simulink library "NHR9400"  (R2020b)
settings: Solver=VariableStepAuto  StartTime=0.0  StopTime=10.0  RelTol=1e-3
undefined symbols (not defined in the file or in its folder): Ts
libraries: simulink x31, fl_lib x19, nesl_utility x12, powerlib_meascontrol x9
settings Model: Creator=argol  LastModifiedBy=argol

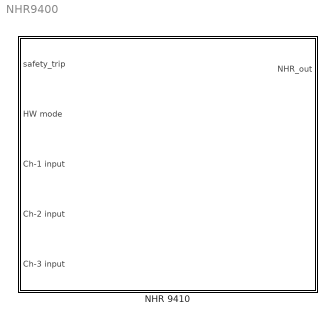
== system NHR9400 ==
  NHR 9410 : Subsystem  mask{p_switch=1, VslewAC=0.0, FslewAC=500.0, VslewDC=0.0, IslewDC=0.0, PslewDC=0.0}
      mask prompts: p_switch "Enter 1 to turn ON, 0 to turn OFF NHR 9410"
      mask DialogControl DescTextVar Prompt: NHR 9410
      mask DialogControl Container3 Prompt: Slew Rates
      mask DialogControl Control2 Prompt: AC Voltage slew rate [0-500000V/s]:
      mask DialogControl f Prompt: Frequency slew rate [0-500 /s]
      mask DialogControl Control3 Prompt: DC Voltage slew rate [0-20000V/s]:
      mask DialogControl Control4 Prompt: DC current slew rate [0-100000A/s]:
      mask DialogControl Control5 Prompt: DC power slew rate [0-1000000W/s]:
      mask Display: image('NHR9410.png');

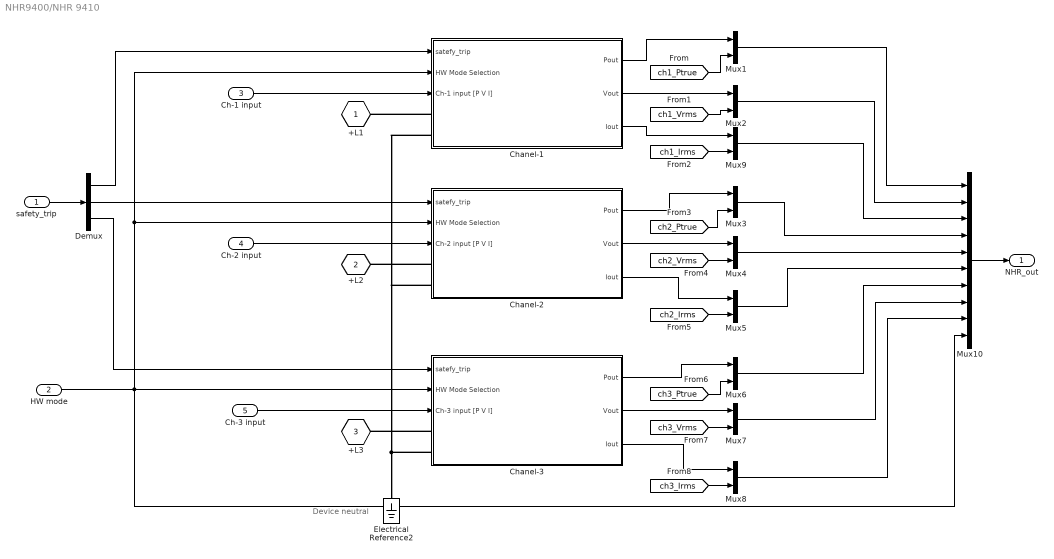
== system NHR9400/NHR 9410 ==
  note: Device neutral
  safety_trip : Inport
  HW mode : Inport  Port=2
  Ch-1 input : Inport  Port=3
  Ch-2 input : Inport  Port=4
  Ch-3 input : Inport  Port=5
  Chanel-1 : Subsystem
  Chanel-2 : Subsystem
  Chanel-3 : Subsystem
  Demux : Demux  Outputs=3
  Electrical Reference2 : fl_lib/Electrical/Electrical Elements/Electrical Reference
  Mux{1..9} (9 alike) : Mux  Inputs=2
  Mux10 : Mux  Inputs=10
  +L1 : PMIOPort  Side=Right
  +L2 : PMIOPort  Port=2  Side=Right
  +L3 : PMIOPort  Port=3  Side=Right
  NHR_out : Outport  VectorParamsAs1DForOutWhenUnconnected=off
  wires:
  Ch-3 input/1 -> Chanel-3/3(Ch-3 input [P V I])
  Ch-1 input/1 -> Chanel-1/3(Ch-1 input [P V I])
  Ch-2 input/1 -> Chanel-2/3(Ch-2 input [P V I])
  Chanel-2/1(Pout) -> Mux3/1
  Chanel-2/2(Vout) -> Mux4/1
  Chanel-2/3(Iout) -> Mux5/1
  Chanel-3/1(Pout) -> Mux6/1
  Chanel-3/2(Vout) -> Mux7/1
  Chanel-3/3(Iout) -> Mux8/1
  [ch2_Ptrue] -> Mux3/2
  [ch2_Vrms] -> Mux4/2
  [ch2_Irms] -> Mux5/2
  [ch3_Ptrue] -> Mux6/2
  [ch3_Vrms] -> Mux7/2
  [ch3_Irms] -> Mux8/2
  Mux1/1 -> Mux10/1
  Mux2/1 -> Mux10/2
  Mux9/1 -> Mux10/3
  Mux3/1 -> Mux10/4
  Mux4/1 -> Mux10/5
  Mux6/1 -> Mux10/7
  Mux7/1 -> Mux10/8
  Mux8/1 -> Mux10/9
  Demux/2 -> Chanel-2/1(satefy_trip)
  Demux/1 -> Chanel-1/1(satefy_trip)
  safety_trip/1 -> Demux/1
  Demux/3 -> Chanel-3/1(satefy_trip)
  Mux5/1 -> Mux10/6
  HW mode/1 -> Chanel-2/2(HW Mode Selection), Chanel-1/2(HW Mode Selection), Mux10/10, Chanel-3/2(HW Mode Selection)
  Mux10/1 -> NHR_out/1
  Chanel-1/2(Vout) -> Mux2/1
  Chanel-1/1(Pout) -> Mux1/1
  Chanel-1/3(Iout) -> Mux9/1
  [ch1_Ptrue] -> Mux1/2
  [ch1_Vrms] -> Mux2/2
  [ch1_Irms] -> Mux9/2
  connections:
  Chanel-1/LConn1 -- +L1/RConn1
  Chanel-2/LConn1 -- +L2/RConn1
  Chanel-3/LConn1 -- +L3/RConn1
  Chanel-3/LConn2 -- Chanel-1/LConn2 -- Chanel-2/LConn2 -- Electrical Reference2/LConn1

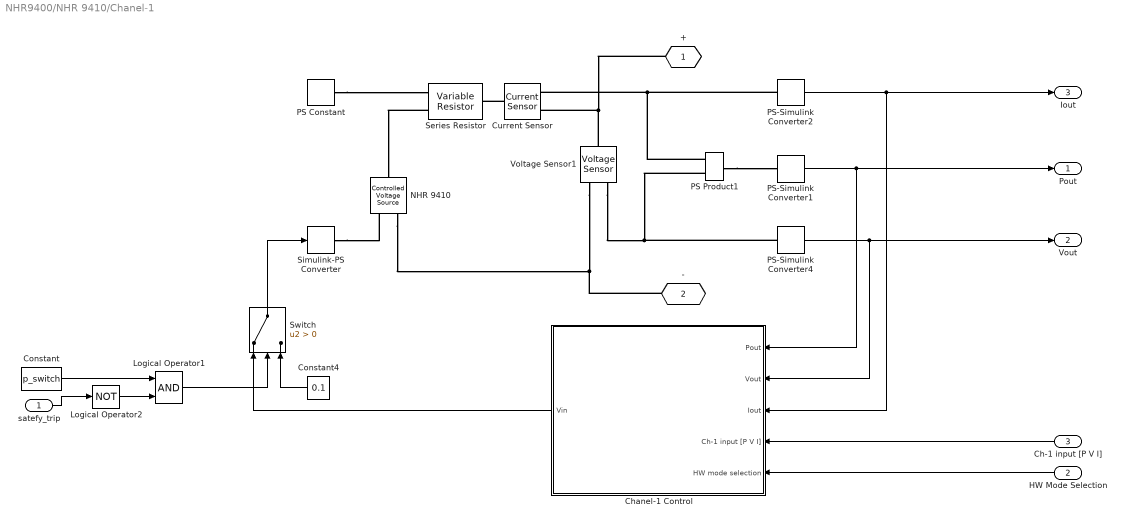
== system NHR9400/NHR 9410/Chanel-1 ==
  satefy_trip : Inport
  HW Mode Selection : Inport  Port=2
  Ch-1 input [P V I] : Inport  Port=3
  Chanel-1 Control : Subsystem
  Constant : Constant  Value=p_switch
  Constant4 : Constant  Value=0.1
  Current Sensor : fl_lib/Electrical/Electrical Sensors/Current Sensor
  Logical Operator1 : Logic  AllPortsSameDT=off  OutDataTypeStr=boolean
  Logical Operator2 : Logic  Operator=NOT  AllPortsSameDT=off  OutDataTypeStr=boolean
  NHR 9410 : fl_lib/Electrical/Electrical Sources/Controlled Voltage Source
  PS Constant : fl_lib/Physical Signals/Sources/PS Constant  constant=0
  PS Product1 : fl_lib/Physical Signals/Functions/PS Product
  PS-Simulink Converter1 : nesl_utility/PS-Simulink Converter  PhysicalDomain=network_engine_domain  SubClassName=ps_output  LeftPortType=input  RightPortType=output  PseudoPeriodic=off  Frequencies=[]  Unit=inherit  AffineConversion=off
  PS-Simulink Converter2 : nesl_utility/PS-Simulink Converter  PhysicalDomain=network_engine_domain  SubClassName=ps_output  LeftPortType=input  RightPortType=output  PseudoPeriodic=off  Frequencies=[]  Unit=1  AffineConversion=off
  PS-Simulink Converter4 : nesl_utility/PS-Simulink Converter  PhysicalDomain=network_engine_domain  SubClassName=ps_output  LeftPortType=input  RightPortType=output  PseudoPeriodic=off  Frequencies=[]  Unit=1  AffineConversion=off
  Series Resistor : fl_lib/Electrical/Electrical Elements/Variable Resistor  Rmin=0.0001 Ohm  i_specify=off  i_priority=None  i=0 A  i_nominal_specify=off  i_nominal_unit=A  i_nominal_value=1  v_specify=off  v_priority=None  v=0 V  v_nominal_specify=off  v_nominal_unit=V  v_nominal_value=1
  Simulink-PS Converter : nesl_utility/Simulink-PS Converter  PhysicalDomain=network_engine_domain  SubClassName=ps_input  LeftPortType=input  RightPortType=output  PseudoPeriodic=off  Frequencies=[]  NoiseDistribution=none  NoiseParameters=[]  Unit=1  AffineConversion=off  FilteringAndDerivatives=filter  SimscapeFilterOrder=1  InputFilterTimeConstant=0.001  UdotUserProvided=0
  Switch : Switch  Criteria=u2 > Threshold  ZeroCross=off
  Voltage Sensor1 : fl_lib/Electrical/Electrical Sensors/Voltage Sensor
  + : PMIOPort  Tag=PMCPort  Side=Left
  - : PMIOPort  Tag=PMCPort  Port=2  Side=Left
  Pout : Outport  VectorParamsAs1DForOutWhenUnconnected=off
  Vout : Outport  Port=2  VectorParamsAs1DForOutWhenUnconnected=off
  Iout : Outport  Port=3  VectorParamsAs1DForOutWhenUnconnected=off
  wires:
  Constant/1 -> Logical Operator1/1
  satefy_trip/1 -> Logical Operator2/1
  Logical Operator2/1 -> Logical Operator1/2
  Switch/1 -> Simulink-PS Converter/1
  Chanel-1 Control/1(Vin) -> Switch/1
  Constant4/1 -> Switch/3
  Logical Operator1/1 -> Switch/2
  PS-Simulink Converter2/1 -> Iout/1, Chanel-1 Control/3(Iout)
  PS-Simulink Converter4/1 -> Vout/1, Chanel-1 Control/2(Vout)
  PS-Simulink Converter1/1 -> Pout/1, Chanel-1 Control/1(Pout)
  HW Mode Selection/1 -> Chanel-1 Control/5(HW mode selection)
  Ch-1 input [P V I]/1 -> Chanel-1 Control/4(Ch-1 input [P V I])
  connections:
  Current Sensor/LConn1 -- Series Resistor/RConn1
  PS Constant/RConn1 -- Series Resistor/LConn1
  PS Product1/RConn1 -- PS-Simulink Converter1/LConn1
  Series Resistor/LConn2 -- NHR 9410/LConn1
  Simulink-PS Converter/RConn1 -- NHR 9410/RConn1
  Voltage Sensor1/LConn1 -- +/RConn1 -- Current Sensor/RConn2
  PS-Simulink Converter2/LConn1 -- PS Product1/LConn1 -- Current Sensor/RConn1
  NHR 9410/RConn2 -- -/RConn1 -- Voltage Sensor1/RConn2
  Voltage Sensor1/RConn1 -- PS Product1/LConn2 -- PS-Simulink Converter4/LConn1

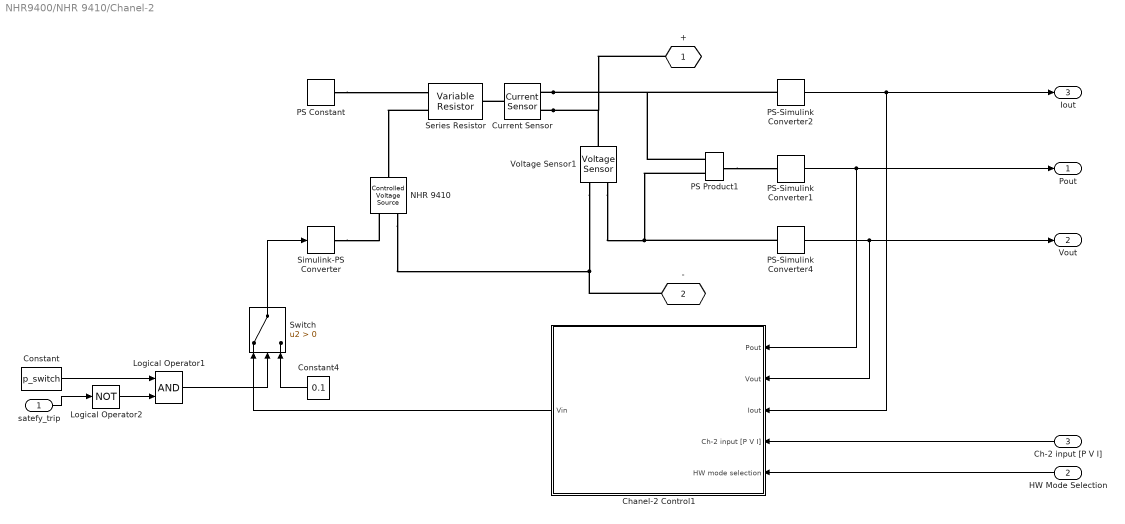
== system NHR9400/NHR 9410/Chanel-2 ==
  satefy_trip : Inport
  HW Mode Selection : Inport  Port=2
  Ch-2 input [P V I] : Inport  Port=3
  Chanel-2 Control1 : Subsystem
  Constant : Constant  Value=p_switch
  Constant4 : Constant  Value=0.1
  Current Sensor : fl_lib/Electrical/Electrical Sensors/Current Sensor
  Logical Operator1 : Logic  AllPortsSameDT=off  OutDataTypeStr=boolean
  Logical Operator2 : Logic  Operator=NOT  AllPortsSameDT=off  OutDataTypeStr=boolean
  NHR 9410 : fl_lib/Electrical/Electrical Sources/Controlled Voltage Source
  PS Constant : fl_lib/Physical Signals/Sources/PS Constant  constant=0
  PS Product1 : fl_lib/Physical Signals/Functions/PS Product
  PS-Simulink Converter1 : nesl_utility/PS-Simulink Converter  PhysicalDomain=network_engine_domain  SubClassName=ps_output  LeftPortType=input  RightPortType=output  PseudoPeriodic=off  Frequencies=[]  Unit=inherit  AffineConversion=off
  PS-Simulink Converter2 : nesl_utility/PS-Simulink Converter  PhysicalDomain=network_engine_domain  SubClassName=ps_output  LeftPortType=input  RightPortType=output  PseudoPeriodic=off  Frequencies=[]  Unit=1  AffineConversion=off
  PS-Simulink Converter4 : nesl_utility/PS-Simulink Converter  PhysicalDomain=network_engine_domain  SubClassName=ps_output  LeftPortType=input  RightPortType=output  PseudoPeriodic=off  Frequencies=[]  Unit=1  AffineConversion=off
  Series Resistor : fl_lib/Electrical/Electrical Elements/Variable Resistor  Rmin=0.0001 Ohm  i_specify=off  i_priority=None  i=0 A  i_nominal_specify=off  i_nominal_unit=A  i_nominal_value=1  v_specify=off  v_priority=None  v=0 V  v_nominal_specify=off  v_nominal_unit=V  v_nominal_value=1
  Simulink-PS Converter : nesl_utility/Simulink-PS Converter  PhysicalDomain=network_engine_domain  SubClassName=ps_input  LeftPortType=input  RightPortType=output  PseudoPeriodic=off  Frequencies=[]  NoiseDistribution=none  NoiseParameters=[]  Unit=1  AffineConversion=off  FilteringAndDerivatives=filter  SimscapeFilterOrder=1  InputFilterTimeConstant=0.001  UdotUserProvided=0
  Switch : Switch  Criteria=u2 > Threshold  ZeroCross=off
  Voltage Sensor1 : fl_lib/Electrical/Electrical Sensors/Voltage Sensor
  + : PMIOPort  Tag=PMCPort  Side=Left
  - : PMIOPort  Tag=PMCPort  Port=2  Side=Left
  Pout : Outport  VectorParamsAs1DForOutWhenUnconnected=off
  Vout : Outport  Port=2  VectorParamsAs1DForOutWhenUnconnected=off
  Iout : Outport  Port=3  VectorParamsAs1DForOutWhenUnconnected=off
  wires:
  Ch-2 input [P V I]/1 -> Chanel-2 Control1/4(Ch-2 input [P V I])
  HW Mode Selection/1 -> Chanel-2 Control1/5(HW mode selection)
  PS-Simulink Converter1/1 -> Chanel-2 Control1/1(Pout), Pout/1
  PS-Simulink Converter4/1 -> Chanel-2 Control1/2(Vout), Vout/1
  PS-Simulink Converter2/1 -> Chanel-2 Control1/3(Iout), Iout/1
  Logical Operator1/1 -> Switch/2
  Constant4/1 -> Switch/3
  Chanel-2 Control1/1(Vin) -> Switch/1
  Switch/1 -> Simulink-PS Converter/1
  Logical Operator2/1 -> Logical Operator1/2
  satefy_trip/1 -> Logical Operator2/1
  Constant/1 -> Logical Operator1/1
  connections:
  PS-Simulink Converter4/LConn1 -- PS Product1/LConn2 -- Voltage Sensor1/RConn1
  Voltage Sensor1/RConn2 -- -/RConn1 -- NHR 9410/RConn2
  Current Sensor/RConn1 -- PS Product1/LConn1 -- PS-Simulink Converter2/LConn1
  Current Sensor/RConn2 -- +/RConn1 -- Voltage Sensor1/LConn1
  Simulink-PS Converter/RConn1 -- NHR 9410/RConn1
  Series Resistor/LConn2 -- NHR 9410/LConn1
  PS Product1/RConn1 -- PS-Simulink Converter1/LConn1
  PS Constant/RConn1 -- Series Resistor/LConn1
  Current Sensor/LConn1 -- Series Resistor/RConn1

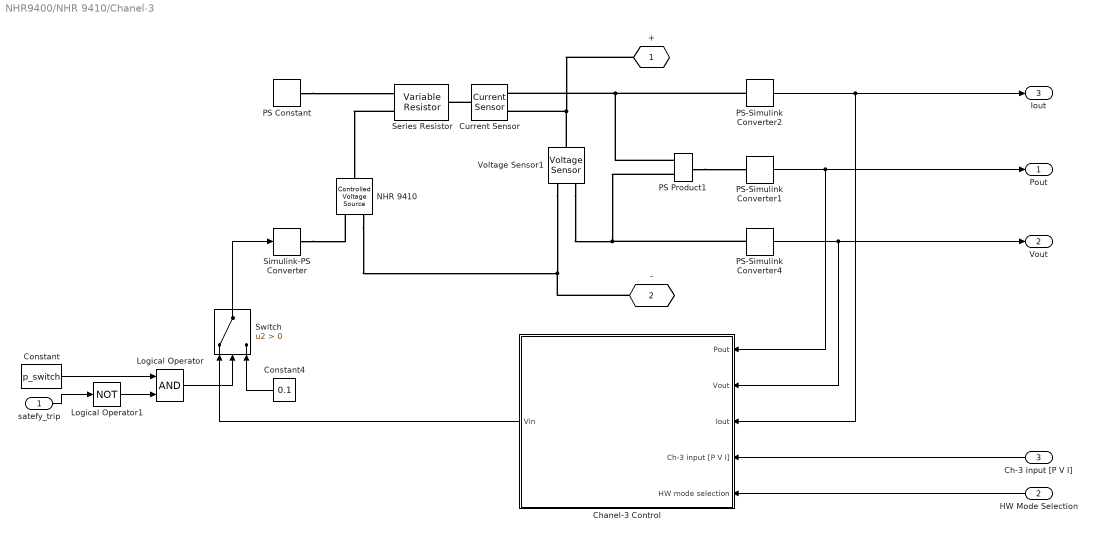
== system NHR9400/NHR 9410/Chanel-3 ==
  satefy_trip : Inport
  HW Mode Selection : Inport  Port=2
  Ch-3 input [P V I] : Inport  Port=3
  Chanel-3 Control : Subsystem
  Constant : Constant  Value=p_switch
  Constant4 : Constant  Value=0.1
  Current Sensor : fl_lib/Electrical/Electrical Sensors/Current Sensor
  Logical Operator : Logic  AllPortsSameDT=off  OutDataTypeStr=boolean
  Logical Operator1 : Logic  Operator=NOT  AllPortsSameDT=off  OutDataTypeStr=boolean
  NHR 9410 : fl_lib/Electrical/Electrical Sources/Controlled Voltage Source
  PS Constant : fl_lib/Physical Signals/Sources/PS Constant  constant=0
  PS Product1 : fl_lib/Physical Signals/Functions/PS Product
  PS-Simulink Converter1 : nesl_utility/PS-Simulink Converter  PhysicalDomain=network_engine_domain  SubClassName=ps_output  LeftPortType=input  RightPortType=output  PseudoPeriodic=off  Frequencies=[]  Unit=inherit  AffineConversion=off
  PS-Simulink Converter2 : nesl_utility/PS-Simulink Converter  PhysicalDomain=network_engine_domain  SubClassName=ps_output  LeftPortType=input  RightPortType=output  PseudoPeriodic=off  Frequencies=[]  Unit=1  AffineConversion=off
  PS-Simulink Converter4 : nesl_utility/PS-Simulink Converter  PhysicalDomain=network_engine_domain  SubClassName=ps_output  LeftPortType=input  RightPortType=output  PseudoPeriodic=off  Frequencies=[]  Unit=1  AffineConversion=off
  Series Resistor : fl_lib/Electrical/Electrical Elements/Variable Resistor  Rmin=0.0001 Ohm  i_specify=off  i_priority=None  i=0 A  i_nominal_specify=off  i_nominal_unit=A  i_nominal_value=1  v_specify=off  v_priority=None  v=0 V  v_nominal_specify=off  v_nominal_unit=V  v_nominal_value=1
  Simulink-PS Converter : nesl_utility/Simulink-PS Converter  PhysicalDomain=network_engine_domain  SubClassName=ps_input  LeftPortType=input  RightPortType=output  PseudoPeriodic=off  Frequencies=[]  NoiseDistribution=none  NoiseParameters=[]  Unit=1  AffineConversion=off  FilteringAndDerivatives=filter  SimscapeFilterOrder=1  InputFilterTimeConstant=0.001  UdotUserProvided=0
  Switch : Switch  Criteria=u2 > Threshold  ZeroCross=off
  Voltage Sensor1 : fl_lib/Electrical/Electrical Sensors/Voltage Sensor
  + : PMIOPort  Tag=PMCPort  Side=Left
  - : PMIOPort  Tag=PMCPort  Port=2  Side=Left
  Pout : Outport  VectorParamsAs1DForOutWhenUnconnected=off
  Vout : Outport  Port=2  VectorParamsAs1DForOutWhenUnconnected=off
  Iout : Outport  Port=3  VectorParamsAs1DForOutWhenUnconnected=off
  wires:
  PS-Simulink Converter2/1 -> Iout/1, Chanel-3 Control/3(Iout)
  PS-Simulink Converter4/1 -> Vout/1, Chanel-3 Control/2(Vout)
  PS-Simulink Converter1/1 -> Pout/1, Chanel-3 Control/1(Pout)
  HW Mode Selection/1 -> Chanel-3 Control/5(HW mode selection)
  Ch-3 input [P V I]/1 -> Chanel-3 Control/4(Ch-3 input [P V I])
  Constant4/1 -> Switch/3
  Chanel-3 Control/1(Vin) -> Switch/1
  Switch/1 -> Simulink-PS Converter/1
  Logical Operator1/1 -> Logical Operator/2
  satefy_trip/1 -> Logical Operator1/1
  Constant/1 -> Logical Operator/1
  Logical Operator/1 -> Switch/2
  connections:
  Current Sensor/LConn1 -- Series Resistor/RConn1
  PS Constant/RConn1 -- Series Resistor/LConn1
  PS Product1/RConn1 -- PS-Simulink Converter1/LConn1
  Series Resistor/LConn2 -- NHR 9410/LConn1
  Simulink-PS Converter/RConn1 -- NHR 9410/RConn1
  Voltage Sensor1/LConn1 -- +/RConn1 -- Current Sensor/RConn2
  PS-Simulink Converter2/LConn1 -- PS Product1/LConn1 -- Current Sensor/RConn1
  NHR 9410/RConn2 -- -/RConn1 -- Voltage Sensor1/RConn2
  Voltage Sensor1/RConn1 -- PS Product1/LConn2 -- PS-Simulink Converter4/LConn1

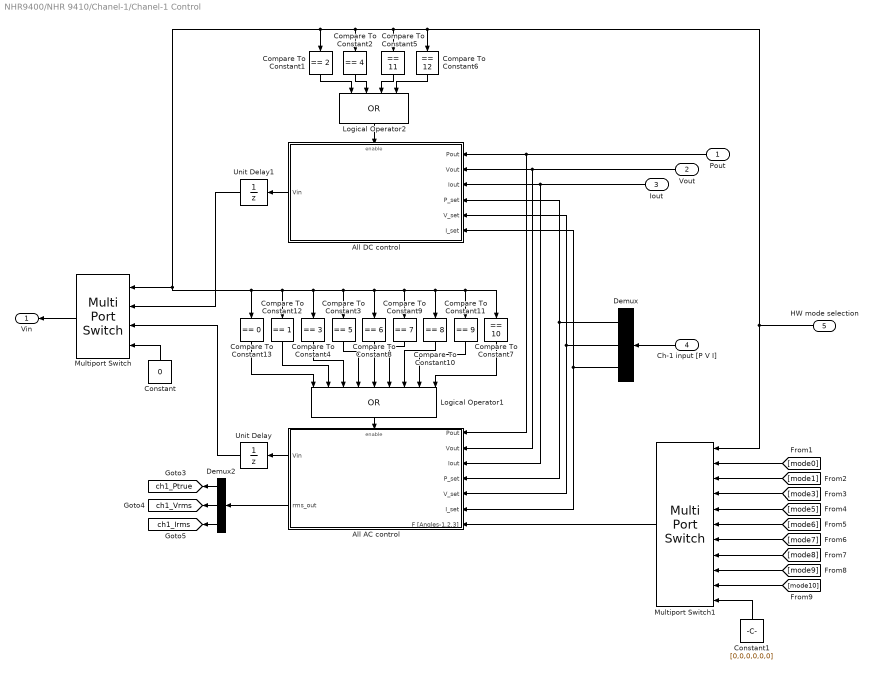
== system NHR9400/NHR 9410/Chanel-1/Chanel-1 Control ==
  Pout : Inport
  Vout : Inport  Port=2
  Iout : Inport  Port=3
  Ch-1 input [P V I] : Inport  Port=4
  HW mode selection : Inport  Port=5
  All AC control : Subsystem
      settings: MinAlgLoopOccurrences=on
  All DC control : Subsystem
      settings: MinAlgLoopOccurrences=on
  Compare To Constant1 : simulink/Logic and Bit Operations/Compare To Constant  relop===  const=2  OutDataTypeStr=boolean
  Compare To Constant10 : simulink/Logic and Bit Operations/Compare To Constant  relop===  const=8  OutDataTypeStr=boolean
  Compare To Constant11 : simulink/Logic and Bit Operations/Compare To Constant  relop===  const=9  OutDataTypeStr=boolean
  Compare To Constant12 : simulink/Logic and Bit Operations/Compare To Constant  relop===  const=1  OutDataTypeStr=boolean
  Compare To Constant13 : simulink/Logic and Bit Operations/Compare To Constant  relop===  const=0  OutDataTypeStr=boolean
  Compare To Constant2 : simulink/Logic and Bit Operations/Compare To Constant  relop===  const=4  OutDataTypeStr=boolean
  Compare To Constant3 : simulink/Logic and Bit Operations/Compare To Constant  relop===  const=5  OutDataTypeStr=boolean
  Compare To Constant4 : simulink/Logic and Bit Operations/Compare To Constant  relop===  const=3  OutDataTypeStr=boolean
  Compare To Constant5 : simulink/Logic and Bit Operations/Compare To Constant  relop===  const=11  OutDataTypeStr=boolean
  Compare To Constant6 : simulink/Logic and Bit Operations/Compare To Constant  relop===  const=12  OutDataTypeStr=boolean
  Compare To Constant7 : simulink/Logic and Bit Operations/Compare To Constant  relop===  const=10  OutDataTypeStr=boolean
  Compare To Constant8 : simulink/Logic and Bit Operations/Compare To Constant  relop===  const=6  OutDataTypeStr=boolean
  Compare To Constant9 : simulink/Logic and Bit Operations/Compare To Constant  relop===  const=7  OutDataTypeStr=boolean
  Constant : Constant  Value=0
  Constant1 : Constant  Value=[0,0,0,0,0,0]
  Demux : Demux  Outputs=3
  Demux2 : Demux  Outputs=3
  Logical Operator1 : Logic  Operator=OR  Inputs=9  AllPortsSameDT=off  OutDataTypeStr=boolean
  Logical Operator2 : Logic  Operator=OR  Inputs=4  AllPortsSameDT=off  OutDataTypeStr=boolean
  Multiport Switch : MultiPortSwitch  DataPortOrder=Specify indices  Inputs=13  DataPortIndices={[2,4,11,12],[0,1,3,5,6,7,8,9,10]}  DataPortForDefault=Additional data port  DiagnosticForDefault=None
  Multiport Switch1 : MultiPortSwitch  DataPortOrder=Specify indices  Inputs=13  DataPortIndices={0,1,3,5,6,7,8,9,10}  DataPortForDefault=Additional data port  DiagnosticForDefault=None
  Unit Delay : UnitDelay  SampleTime=-1  HasFrameUpgradeWarning=on
  Unit Delay1 : UnitDelay  SampleTime=-1  HasFrameUpgradeWarning=on
  Vin : Outport  VectorParamsAs1DForOutWhenUnconnected=off
  tag scope: ch1_Irms=global, ch1_Ptrue=global, ch1_Vrms=global
  wires:
  Compare To Constant2/1 -> Logical Operator2/2
  Compare To Constant1/1 -> Logical Operator2/1
  HW mode selection/1 -> Multiport Switch1/1, Compare To Constant6/1, Compare To Constant5/1, Compare To Constant2/1, Compare To Constant1/1, Multiport Switch/1, Compare To Constant13/1, Compare To Constant12/1, Compare To Constant3/1, Compare To Constant7/1, Compare To Constant11/1, Compare To Constant10/1, Compare To Constant9/1, Compare To Constant8/1, Compare To Constant4/1
  All AC control/1(Vin) -> Unit Delay/1
  All DC control/1(Vin) -> Unit Delay1/1
  All AC control/2(rms_out) -> Demux2/1
  Logical Operator1/1 -> All AC control/Enable
  Logical Operator2/1 -> All DC control/Enable
  Constant/1 -> Multiport Switch/4
  Multiport Switch/1 -> Vin/1
  Pout/1 -> All DC control/1(Pout), All AC control/1(Pout)
  Iout/1 -> All DC control/3(Iout), All AC control/3(Iout)
  Demux2/1 -> [ch1_Ptrue]
  Demux2/3 -> [ch1_Irms]
  Demux2/2 -> [ch1_Vrms]
  Vout/1 -> All DC control/2(Vout), All AC control/2(Vout)
  Ch-1 input [P V I]/1 -> Demux/1
  Demux/1 -> All AC control/4(P_set), All DC control/4(P_set)
  Demux/2 -> All AC control/5(V_set), All DC control/5(V_set)
  Demux/3 -> All AC control/6(I_set), All DC control/6(I_set)
  Compare To Constant5/1 -> Logical Operator2/3
  Compare To Constant6/1 -> Logical Operator2/4
  Compare To Constant8/1 -> Logical Operator1/5
  Compare To Constant9/1 -> Logical Operator1/6
  Compare To Constant10/1 -> Logical Operator1/7
  Compare To Constant11/1 -> Logical Operator1/8
  Compare To Constant7/1 -> Logical Operator1/9
  Compare To Constant13/1 -> Logical Operator1/1
  Compare To Constant12/1 -> Logical Operator1/2
  Compare To Constant4/1 -> Logical Operator1/3
  Compare To Constant3/1 -> Logical Operator1/4
  [mode0] -> Multiport Switch1/2
  [mode1] -> Multiport Switch1/3
  [mode3] -> Multiport Switch1/4
  [mode5] -> Multiport Switch1/5
  [mode6] -> Multiport Switch1/6
  [mode7] -> Multiport Switch1/7
  [mode8] -> Multiport Switch1/8
  [mode9] -> Multiport Switch1/9
  [mode10] -> Multiport Switch1/10
  Constant1/1 -> Multiport Switch1/11
  Multiport Switch1/1 -> All AC control/7(F [Angles-1,2,3])
  Unit Delay/1 -> Multiport Switch/3
  Unit Delay1/1 -> Multiport Switch/2

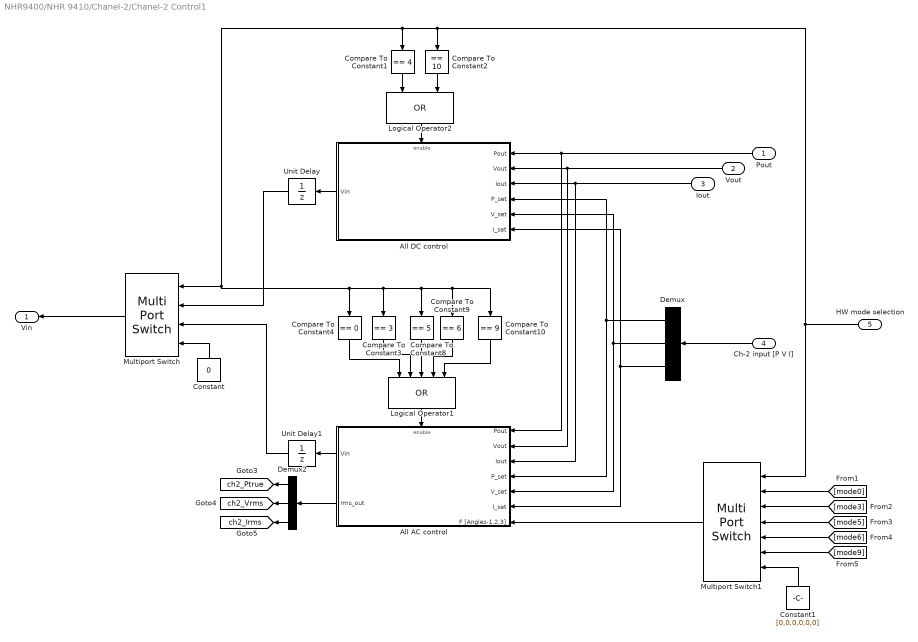
== system NHR9400/NHR 9410/Chanel-2/Chanel-2 Control1 ==
  Pout : Inport
  Vout : Inport  Port=2
  Iout : Inport  Port=3
  Ch-2 input [P V I] : Inport  Port=4
  HW mode selection : Inport  Port=5
  All AC control : Subsystem
      settings: MinAlgLoopOccurrences=on
  All DC control : Subsystem
      settings: MinAlgLoopOccurrences=on
  Compare To Constant1 : simulink/Logic and Bit Operations/Compare To Constant  relop===  const=4  OutDataTypeStr=boolean
  Compare To Constant10 : simulink/Logic and Bit Operations/Compare To Constant  relop===  const=9  OutDataTypeStr=boolean
  Compare To Constant2 : simulink/Logic and Bit Operations/Compare To Constant  relop===  const=10  OutDataTypeStr=boolean
  Compare To Constant3 : simulink/Logic and Bit Operations/Compare To Constant  relop===  const=3  OutDataTypeStr=boolean
  Compare To Constant4 : simulink/Logic and Bit Operations/Compare To Constant  relop===  const=0  OutDataTypeStr=boolean
  Compare To Constant8 : simulink/Logic and Bit Operations/Compare To Constant  relop===  const=5  OutDataTypeStr=boolean
  Compare To Constant9 : simulink/Logic and Bit Operations/Compare To Constant  relop===  const=6  OutDataTypeStr=boolean
  Constant : Constant  Value=0
  Constant1 : Constant  Value=[0,0,0,0,0,0]
  Demux : Demux  Outputs=3
  Demux2 : Demux  Outputs=3
  Logical Operator1 : Logic  Operator=OR  Inputs=5  AllPortsSameDT=off  OutDataTypeStr=boolean
  Logical Operator2 : Logic  Operator=OR  AllPortsSameDT=off  OutDataTypeStr=boolean
  Multiport Switch : MultiPortSwitch  DataPortOrder=Specify indices  Inputs=13  DataPortIndices={[4,10],[0,3,5,6,9]}  DataPortForDefault=Additional data port  DiagnosticForDefault=None
  Multiport Switch1 : MultiPortSwitch  DataPortOrder=Specify indices  Inputs=13  DataPortIndices={0,3,5,6,9}  DataPortForDefault=Additional data port  DiagnosticForDefault=None
  Unit Delay : UnitDelay  SampleTime=-1  HasFrameUpgradeWarning=on
  Unit Delay1 : UnitDelay  SampleTime=-1  HasFrameUpgradeWarning=on
  Vin : Outport  VectorParamsAs1DForOutWhenUnconnected=off
  tag scope: ch2_Irms=global, ch2_Ptrue=global, ch2_Vrms=global
  wires:
  Demux/3 -> All DC control/6(I_set), All AC control/6(I_set)
  Demux/2 -> All DC control/5(V_set), All AC control/5(V_set)
  Demux/1 -> All DC control/4(P_set), All AC control/4(P_set)
  Ch-2 input [P V I]/1 -> Demux/1
  Vout/1 -> All DC control/2(Vout), All AC control/2(Vout)
  Demux2/2 -> [ch2_Vrms]
  Demux2/3 -> [ch2_Irms]
  Demux2/1 -> [ch2_Ptrue]
  Iout/1 -> All DC control/3(Iout), All AC control/3(Iout)
  Pout/1 -> All DC control/1(Pout), All AC control/1(Pout)
  Multiport Switch/1 -> Vin/1
  Constant/1 -> Multiport Switch/4
  Logical Operator2/1 -> All DC control/Enable
  Compare To Constant4/1 -> Logical Operator1/1
  Compare To Constant3/1 -> Logical Operator1/2
  Compare To Constant8/1 -> Logical Operator1/3
  Compare To Constant9/1 -> Logical Operator1/4
  Compare To Constant10/1 -> Logical Operator1/5
  Logical Operator1/1 -> All AC control/Enable
  All AC control/2(rms_out) -> Demux2/1
  All DC control/1(Vin) -> Unit Delay/1
  All AC control/1(Vin) -> Unit Delay1/1
  Multiport Switch1/1 -> All AC control/7(F [Angles-1,2,3])
  HW mode selection/1 -> Compare To Constant4/1, Compare To Constant10/1, Compare To Constant9/1, Compare To Constant8/1, Compare To Constant3/1, Multiport Switch/1, Compare To Constant1/1, Compare To Constant2/1, Multiport Switch1/1
  [mode0] -> Multiport Switch1/2
  [mode3] -> Multiport Switch1/3
  [mode5] -> Multiport Switch1/4
  [mode6] -> Multiport Switch1/5
  [mode9] -> Multiport Switch1/6
  Constant1/1 -> Multiport Switch1/7
  Compare To Constant1/1 -> Logical Operator2/1
  Compare To Constant2/1 -> Logical Operator2/2
  Unit Delay/1 -> Multiport Switch/2
  Unit Delay1/1 -> Multiport Switch/3

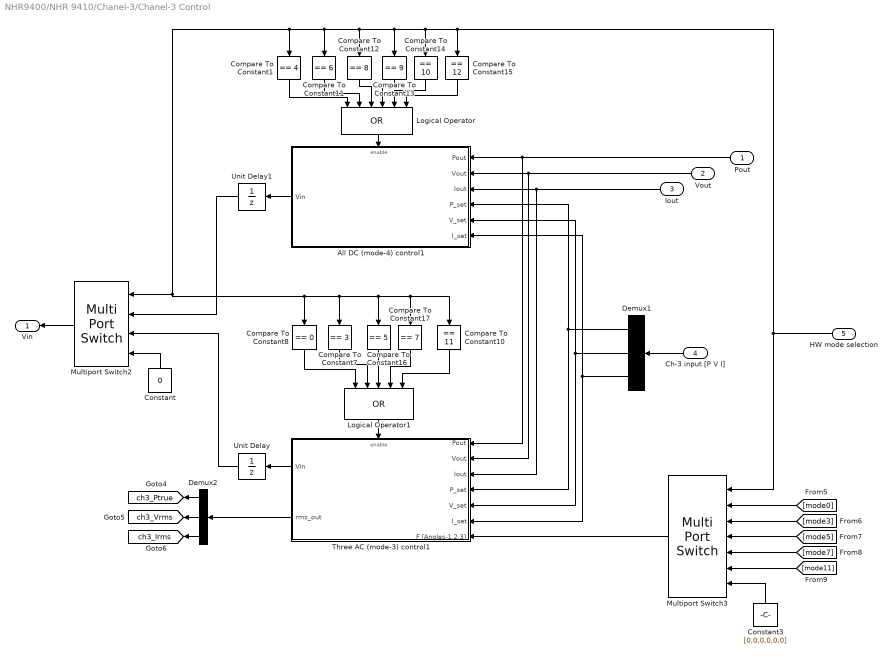
== system NHR9400/NHR 9410/Chanel-3/Chanel-3 Control ==
  Pout : Inport
  Vout : Inport  Port=2
  Iout : Inport  Port=3
  Ch-3 input [P V I] : Inport  Port=4
  HW mode selection : Inport  Port=5
  All DC (mode-4) control1 : Subsystem
      settings: MinAlgLoopOccurrences=on
  Compare To Constant1 : simulink/Logic and Bit Operations/Compare To Constant  relop===  const=4  OutDataTypeStr=boolean
  Compare To Constant10 : simulink/Logic and Bit Operations/Compare To Constant  relop===  const=11  OutDataTypeStr=boolean
  Compare To Constant11 : simulink/Logic and Bit Operations/Compare To Constant  relop===  const=6  OutDataTypeStr=boolean
  Compare To Constant12 : simulink/Logic and Bit Operations/Compare To Constant  relop===  const=8  OutDataTypeStr=boolean
  Compare To Constant13 : simulink/Logic and Bit Operations/Compare To Constant  relop===  const=9  OutDataTypeStr=boolean
  Compare To Constant14 : simulink/Logic and Bit Operations/Compare To Constant  relop===  const=10  OutDataTypeStr=boolean
  Compare To Constant15 : simulink/Logic and Bit Operations/Compare To Constant  relop===  const=12  OutDataTypeStr=boolean
  Compare To Constant16 : simulink/Logic and Bit Operations/Compare To Constant  relop===  const=5  OutDataTypeStr=boolean
  Compare To Constant17 : simulink/Logic and Bit Operations/Compare To Constant  relop===  const=7  OutDataTypeStr=boolean
  Compare To Constant7 : simulink/Logic and Bit Operations/Compare To Constant  relop===  const=3  OutDataTypeStr=boolean
  Compare To Constant8 : simulink/Logic and Bit Operations/Compare To Constant  relop===  const=0  OutDataTypeStr=boolean
  Constant : Constant  Value=0
  Constant3 : Constant  Value=[0,0,0,0,0,0]
  Demux1 : Demux  Outputs=3
  Demux2 : Demux  Outputs=3
  Logical Operator : Logic  Operator=OR  Inputs=6  AllPortsSameDT=off  OutDataTypeStr=boolean
  Logical Operator1 : Logic  Operator=OR  Inputs=5  AllPortsSameDT=off  OutDataTypeStr=boolean
  Multiport Switch2 : MultiPortSwitch  DataPortOrder=Specify indices  Inputs=13  DataPortIndices={[4,6,8,9,10,12],[0,3,5,7,11]}  DataPortForDefault=Additional data port  DiagnosticForDefault=None
  Multiport Switch3 : MultiPortSwitch  DataPortOrder=Specify indices  Inputs=13  DataPortIndices={0,3,5,7,11}  DataPortForDefault=Additional data port  DiagnosticForDefault=None
  Three AC (mode-3) control1 : Subsystem
      settings: MinAlgLoopOccurrences=on
  Unit Delay : UnitDelay  SampleTime=-1  HasFrameUpgradeWarning=on
  Unit Delay1 : UnitDelay  SampleTime=-1  HasFrameUpgradeWarning=on
  Vin : Outport  VectorParamsAs1DForOutWhenUnconnected=off
  tag scope: ch3_Irms=global, ch3_Ptrue=global, ch3_Vrms=global
  wires:
  Demux2/2 -> [ch3_Vrms]
  Demux2/3 -> [ch3_Irms]
  Demux2/1 -> [ch3_Ptrue]
  Multiport Switch3/1 -> Three AC (mode-3) control1/7(F [Angles-1,2,3])
  Compare To Constant17/1 -> Logical Operator1/4
  Iout/1 -> All DC (mode-4) control1/3(Iout), Three AC (mode-3) control1/3(Iout)
  Three AC (mode-3) control1/1(Vin) -> Unit Delay/1
  Multiport Switch2/1 -> Vin/1
  [mode11] -> Multiport Switch3/6
  Logical Operator1/1 -> Three AC (mode-3) control1/Enable
  Demux1/1 -> All DC (mode-4) control1/4(P_set), Three AC (mode-3) control1/4(P_set)
  Compare To Constant10/1 -> Logical Operator1/5
  [mode0] -> Multiport Switch3/2
  Compare To Constant8/1 -> Logical Operator1/1
  Demux1/2 -> All DC (mode-4) control1/5(V_set), Three AC (mode-3) control1/5(V_set)
  Pout/1 -> All DC (mode-4) control1/1(Pout), Three AC (mode-3) control1/1(Pout)
  Demux1/3 -> All DC (mode-4) control1/6(I_set), Three AC (mode-3) control1/6(I_set)
  Vout/1 -> All DC (mode-4) control1/2(Vout), Three AC (mode-3) control1/2(Vout)
  [mode5] -> Multiport Switch3/4
  Ch-3 input [P V I]/1 -> Demux1/1
  [mode3] -> Multiport Switch3/3
  [mode7] -> Multiport Switch3/5
  Compare To Constant16/1 -> Logical Operator1/3
  All DC (mode-4) control1/1(Vin) -> Unit Delay1/1
  Constant3/1 -> Multiport Switch3/7
  Compare To Constant7/1 -> Logical Operator1/2
  Constant/1 -> Multiport Switch2/4
  Three AC (mode-3) control1/2(rms_out) -> Demux2/1
  Logical Operator/1 -> All DC (mode-4) control1/Enable
  Compare To Constant15/1 -> Logical Operator/6
  Compare To Constant14/1 -> Logical Operator/5
  Compare To Constant13/1 -> Logical Operator/4
  Compare To Constant1/1 -> Logical Operator/1
  Compare To Constant11/1 -> Logical Operator/2
  HW mode selection/1 -> Compare To Constant8/1, Compare To Constant10/1, Compare To Constant17/1, Compare To Constant16/1, Compare To Constant7/1, Multiport Switch2/1, Compare To Constant1/1, Compare To Constant11/1, Compare To Constant12/1, Compare To Constant13/1, Compare To Constant14/1, Compare To Constant15/1, Multiport Switch3/1
  Compare To Constant12/1 -> Logical Operator/3
  Unit Delay/1 -> Multiport Switch2/3
  Unit Delay1/1 -> Multiport Switch2/2

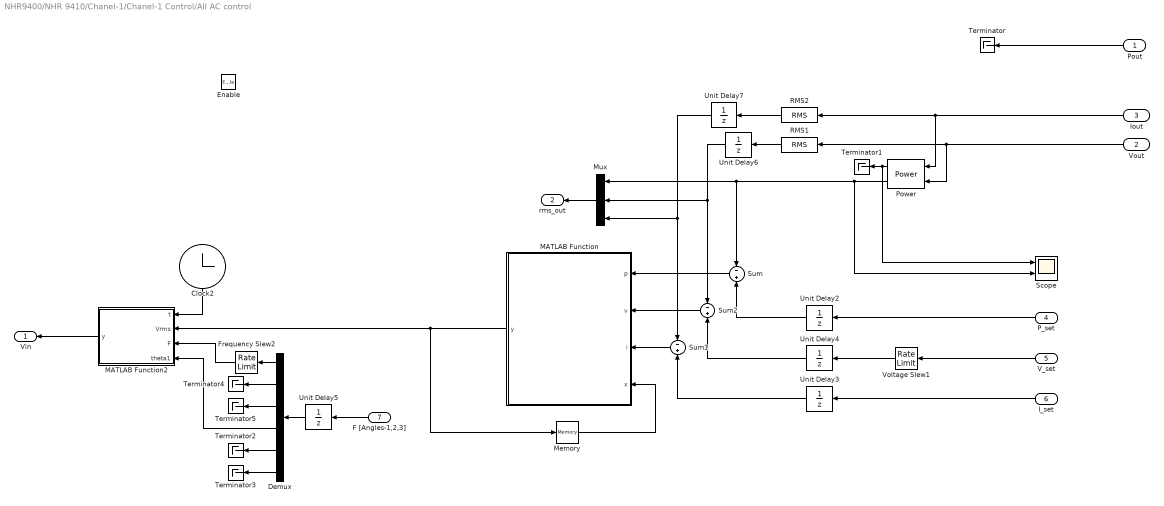
== system NHR9400/NHR 9410/Chanel-1/Chanel-1 Control/All AC control ==
  Pout : Inport
  Vout : Inport  Port=2
  Iout : Inport  Port=3
  P_set : Inport  Port=4
  V_set : Inport  Port=5
  I_set : Inport  Port=6
  F [Angles-1,2,3] : Inport  Port=7
  Enable : EnablePort
  Clock2 : Clock
  Demux : Demux  Outputs=6
  Frequency Slew2 : RateLimiter  RisingSlewLimit=FslewAC  FallingSlewLimit=-FslewAC  SampleTimeMode=inherited  LinearizeAsGain=off
  MATLAB Function : MATLAB Function  TreatAsAtomicUnit=on
  MATLAB Function2 : MATLAB Function  TreatAsAtomicUnit=on
  Memory : Memory
  Mux : Mux  Inputs=3
  Power : powerlib_meascontrol/Measurements/Power  Freq=60  Vinit=[0, 0]  Iinit=[0, 0]  Ts=Ts
  RMS1 : powerlib_meascontrol/Measurements/RMS  TrueRMS=on  Freq=60  RMSInit=0  Ts=0
  RMS2 : powerlib_meascontrol/Measurements/RMS  TrueRMS=on  Freq=60  RMSInit=0  Ts=0
  Scope : Scope  NumInputPorts=2
  Sum : Sum  Inputs=-+
  Sum1 : Sum  Inputs=-+
  Sum2 : Sum  Inputs=-+
  Terminator{,1..5} (6 alike) : Terminator
  Unit Delay{2..7} (6 alike) : UnitDelay  SampleTime=-1  HasFrameUpgradeWarning=on
  Voltage Slew1 : RateLimiter  RisingSlewLimit=VslewAC  FallingSlewLimit=-VslewAC  SampleTimeMode=inherited  LinearizeAsGain=off
  Vin : Outport  VectorParamsAs1DForOutWhenUnconnected=off
  rms_out : Outport  Port=2  VectorParamsAs1DForOutWhenUnconnected=off
  wires:
  Voltage Slew1/1 -> Unit Delay4/1
  Frequency Slew2/1 -> MATLAB Function2/3(F)
  F [Angles-1,2,3]/1 -> Unit Delay5/1
  Demux/6 -> Terminator3/1
  Demux/3 -> Terminator5/1
  Mux/1 -> rms_out/1
  Power/1 -> Scope/2, Sum/1, Mux/1
  MATLAB Function2/1(y) -> Vin/1
  Clock2/1 -> MATLAB Function2/1(t)
  Memory/1 -> MATLAB Function/4(x)
  RMS2/1 -> Unit Delay7/1
  RMS1/1 -> Unit Delay6/1
  P_set/1 -> Unit Delay2/1
  I_set/1 -> Unit Delay3/1
  Sum1/1 -> MATLAB Function/3(i)
  Sum2/1 -> MATLAB Function/2(v)
  Sum/1 -> MATLAB Function/1(p)
  Power/2 -> Scope/1, Terminator1/1
  Pout/1 -> Terminator/1
  Demux/1 -> Frequency Slew2/1
  Demux/2 -> Terminator4/1
  Demux/5 -> Terminator2/1
  Demux/4 -> MATLAB Function2/4(theta1)
  MATLAB Function/1(y) -> Memory/1, MATLAB Function2/2(Vrms)
  Vout/1 -> Power/1, RMS1/1
  Iout/1 -> Power/2, RMS2/1
  Unit Delay2/1 -> Sum/2
  Unit Delay3/1 -> Sum1/2
  V_set/1 -> Voltage Slew1/1
  Unit Delay4/1 -> Sum2/2
  Unit Delay5/1 -> Demux/1
  Unit Delay6/1 -> Sum2/1, Mux/2
  Unit Delay7/1 -> Sum1/1, Mux/3

== system NHR9400/NHR 9410/Chanel-1/Chanel-1 Control/All DC control ==
  Pout : Inport
  Vout : Inport  Port=2
  Iout : Inport  Port=3
  P_set : Inport  Port=4
  V_set : Inport  Port=5
  I_set : Inport  Port=6
  Enable : EnablePort
  Current Slew : RateLimiter  RisingSlewLimit=IslewDC  FallingSlewLimit=-IslewDC  SampleTimeMode=inherited  LinearizeAsGain=off
  MATLAB Function : MATLAB Function  TreatAsAtomicUnit=on
  Memory : Memory
  Power Slew : RateLimiter  RisingSlewLimit=PslewDC  FallingSlewLimit=-PslewDC  SampleTimeMode=inherited  LinearizeAsGain=off
  Sum : Sum  Inputs=-+
  Sum1 : Sum  Inputs=-+
  Sum2 : Sum  Inputs=-+
  Unit Delay{,1..5} (6 alike) : UnitDelay  SampleTime=-1  HasFrameUpgradeWarning=on
  Voltage Slew : RateLimiter  RisingSlewLimit=VslewDC  FallingSlewLimit=-VslewDC  SampleTimeMode=inherited  LinearizeAsGain=off
  Vin : Outport  VectorParamsAs1DForOutWhenUnconnected=off
  wires:
  Power Slew/1 -> Unit Delay4/1
  Voltage Slew/1 -> Unit Delay3/1
  Current Slew/1 -> Unit Delay5/1
  I_set/1 -> Current Slew/1
  V_set/1 -> Voltage Slew/1
  P_set/1 -> Power Slew/1
  MATLAB Function/1(y) -> Memory/1, Vin/1
  Sum/1 -> MATLAB Function/1(p)
  Sum1/1 -> MATLAB Function/3(i)
  Sum2/1 -> MATLAB Function/2(v)
  Memory/1 -> MATLAB Function/4(x)
  Unit Delay2/1 -> Sum/1
  Vout/1 -> Unit Delay1/1
  Unit Delay/1 -> Sum1/1
  Unit Delay1/1 -> Sum2/1
  Unit Delay3/1 -> Sum2/2
  Unit Delay4/1 -> Sum/2
  Unit Delay5/1 -> Sum1/2
  Iout/1 -> Unit Delay/1
  Pout/1 -> Unit Delay2/1

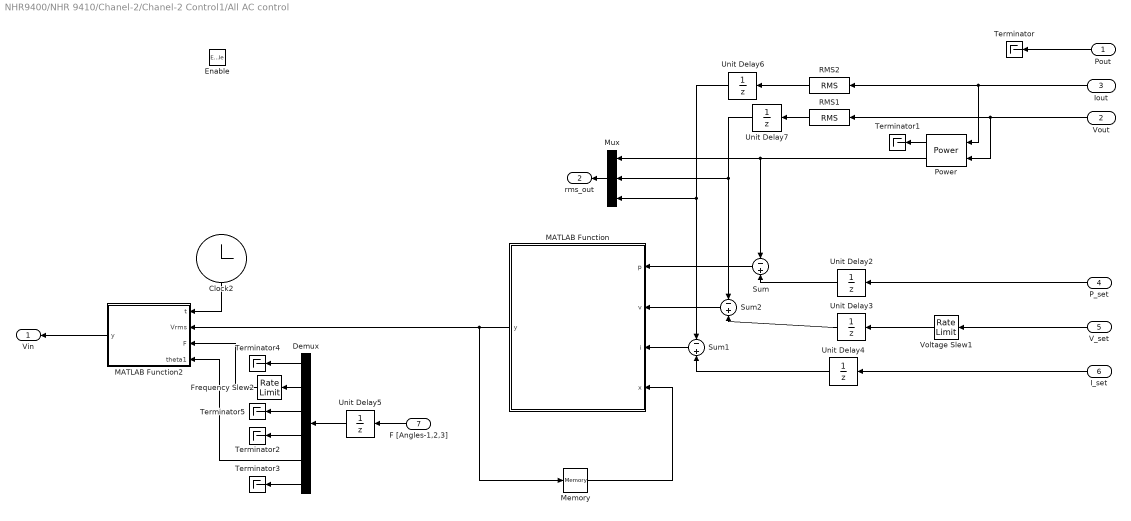
== system NHR9400/NHR 9410/Chanel-2/Chanel-2 Control1/All AC control ==
  Pout : Inport
  Vout : Inport  Port=2
  Iout : Inport  Port=3
  P_set : Inport  Port=4
  V_set : Inport  Port=5
  I_set : Inport  Port=6
  F [Angles-1,2,3] : Inport  Port=7
  Enable : EnablePort
  Clock2 : Clock
  Demux : Demux  Outputs=6
  Frequency Slew2 : RateLimiter  RisingSlewLimit=FslewAC  FallingSlewLimit=-FslewAC  SampleTimeMode=inherited  LinearizeAsGain=off
  MATLAB Function : MATLAB Function  TreatAsAtomicUnit=on
  MATLAB Function2 : MATLAB Function  TreatAsAtomicUnit=on
  Memory : Memory
  Mux : Mux  Inputs=3
  Power : powerlib_meascontrol/Measurements/Power  Freq=60  Vinit=[0, 0]  Iinit=[0, 0]  Ts=0
  RMS1 : powerlib_meascontrol/Measurements/RMS  TrueRMS=on  Freq=60  RMSInit=0  Ts=0
  RMS2 : powerlib_meascontrol/Measurements/RMS  TrueRMS=on  Freq=60  RMSInit=0  Ts=0
  Sum : Sum  Inputs=-+
  Sum1 : Sum  Inputs=-+
  Sum2 : Sum  Inputs=-+
  Terminator{,1..5} (6 alike) : Terminator
  Unit Delay{2..7} (6 alike) : UnitDelay  SampleTime=-1  HasFrameUpgradeWarning=on
  Voltage Slew1 : RateLimiter  RisingSlewLimit=VslewAC  FallingSlewLimit=-VslewAC  SampleTimeMode=inherited  LinearizeAsGain=off
  Vin : Outport  VectorParamsAs1DForOutWhenUnconnected=off
  rms_out : Outport  Port=2  VectorParamsAs1DForOutWhenUnconnected=off
  wires:
  MATLAB Function/1(y) -> MATLAB Function2/2(Vrms), Memory/1
  Pout/1 -> Terminator/1
  Power/2 -> Terminator1/1
  Sum/1 -> MATLAB Function/1(p)
  Sum2/1 -> MATLAB Function/2(v)
  Sum1/1 -> MATLAB Function/3(i)
  I_set/1 -> Unit Delay4/1
  P_set/1 -> Unit Delay2/1
  RMS1/1 -> Unit Delay7/1
  RMS2/1 -> Unit Delay6/1
  Memory/1 -> MATLAB Function/4(x)
  Clock2/1 -> MATLAB Function2/1(t)
  MATLAB Function2/1(y) -> Vin/1
  Power/1 -> Sum/1, Mux/1
  Mux/1 -> rms_out/1
  Demux/3 -> Terminator5/1
  Demux/6 -> Terminator3/1
  F [Angles-1,2,3]/1 -> Unit Delay5/1
  Demux/1 -> Terminator4/1
  Demux/4 -> Terminator2/1
  Demux/5 -> MATLAB Function2/4(theta1)
  V_set/1 -> Voltage Slew1/1
  Demux/2 -> Frequency Slew2/1
  Frequency Slew2/1 -> MATLAB Function2/3(F)
  Voltage Slew1/1 -> Unit Delay3/1
  Iout/1 -> RMS2/1, Power/2
  Vout/1 -> RMS1/1, Power/1
  Unit Delay2/1 -> Sum/2
  Unit Delay3/1 -> Sum2/2
  Unit Delay4/1 -> Sum1/2
  Unit Delay5/1 -> Demux/1
  Unit Delay6/1 -> Sum1/1, Mux/3
  Unit Delay7/1 -> Sum2/1, Mux/2

== system NHR9400/NHR 9410/Chanel-2/Chanel-2 Control1/All DC control ==
  Pout : Inport
  Vout : Inport  Port=2
  Iout : Inport  Port=3
  P_set : Inport  Port=4
  V_set : Inport  Port=5
  I_set : Inport  Port=6
  Enable : EnablePort
  Current Slew : RateLimiter  RisingSlewLimit=IslewDC  FallingSlewLimit=-IslewDC  SampleTimeMode=inherited  LinearizeAsGain=off
  MATLAB Function : MATLAB Function  TreatAsAtomicUnit=on
  Memory : Memory
  Power Slew : RateLimiter  RisingSlewLimit=PslewDC  FallingSlewLimit=-PslewDC  SampleTimeMode=inherited  LinearizeAsGain=off
  Sum : Sum  Inputs=-+
  Sum1 : Sum  Inputs=-+
  Sum2 : Sum  Inputs=-+
  Unit Delay{1..3,5..7} (6 alike) : UnitDelay  SampleTime=-1  HasFrameUpgradeWarning=on
  Voltage Slew : RateLimiter  RisingSlewLimit=VslewDC  FallingSlewLimit=-VslewDC  SampleTimeMode=inherited  LinearizeAsGain=off
  Vin : Outport  VectorParamsAs1DForOutWhenUnconnected=off
  wires:
  Memory/1 -> MATLAB Function/4(x)
  Sum2/1 -> MATLAB Function/2(v)
  Sum1/1 -> MATLAB Function/3(i)
  Sum/1 -> MATLAB Function/1(p)
  MATLAB Function/1(y) -> Vin/1, Memory/1
  P_set/1 -> Power Slew/1
  V_set/1 -> Voltage Slew/1
  I_set/1 -> Current Slew/1
  Current Slew/1 -> Unit Delay7/1
  Voltage Slew/1 -> Unit Delay6/1
  Power Slew/1 -> Unit Delay5/1
  Unit Delay2/1 -> Sum/1
  Vout/1 -> Unit Delay1/1
  Unit Delay3/1 -> Sum1/1
  Unit Delay1/1 -> Sum2/1
  Unit Delay5/1 -> Sum/2
  Unit Delay6/1 -> Sum2/2
  Unit Delay7/1 -> Sum1/2
  Iout/1 -> Unit Delay3/1
  Pout/1 -> Unit Delay2/1

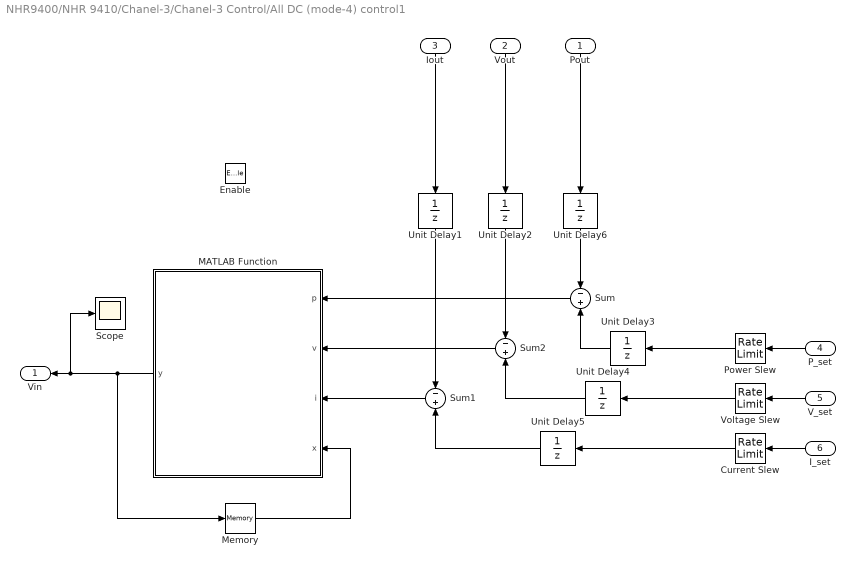
== system NHR9400/NHR 9410/Chanel-3/Chanel-3 Control/All DC (mode-4) control1 ==
  Pout : Inport
  Vout : Inport  Port=2
  Iout : Inport  Port=3
  P_set : Inport  Port=4
  V_set : Inport  Port=5
  I_set : Inport  Port=6
  Enable : EnablePort
  Current Slew : RateLimiter  RisingSlewLimit=IslewDC  FallingSlewLimit=-IslewDC  SampleTimeMode=inherited  LinearizeAsGain=off
  MATLAB Function : MATLAB Function  TreatAsAtomicUnit=on
  Memory : Memory
  Power Slew : RateLimiter  RisingSlewLimit=PslewDC  FallingSlewLimit=-PslewDC  SampleTimeMode=inherited  LinearizeAsGain=off
  Scope : Scope
  Sum : Sum  Inputs=-+
  Sum1 : Sum  Inputs=-+
  Sum2 : Sum  Inputs=-+
  Unit Delay{1..6} (6 alike) : UnitDelay  SampleTime=-1  HasFrameUpgradeWarning=on
  Voltage Slew : RateLimiter  RisingSlewLimit=VslewDC  FallingSlewLimit=-VslewDC  SampleTimeMode=inherited  LinearizeAsGain=off
  Vin : Outport  VectorParamsAs1DForOutWhenUnconnected=off
  wires:
  Memory/1 -> MATLAB Function/4(x)
  Sum2/1 -> MATLAB Function/2(v)
  Sum1/1 -> MATLAB Function/3(i)
  Sum/1 -> MATLAB Function/1(p)
  MATLAB Function/1(y) -> Scope/1, Vin/1, Memory/1
  P_set/1 -> Power Slew/1
  V_set/1 -> Voltage Slew/1
  I_set/1 -> Current Slew/1
  Current Slew/1 -> Unit Delay5/1
  Voltage Slew/1 -> Unit Delay4/1
  Power Slew/1 -> Unit Delay3/1
  Unit Delay1/1 -> Sum1/1
  Vout/1 -> Unit Delay2/1
  Unit Delay6/1 -> Sum/1
  Unit Delay3/1 -> Sum/2
  Unit Delay4/1 -> Sum2/2
  Unit Delay5/1 -> Sum1/2
  Unit Delay2/1 -> Sum2/1
  Iout/1 -> Unit Delay1/1
  Pout/1 -> Unit Delay6/1

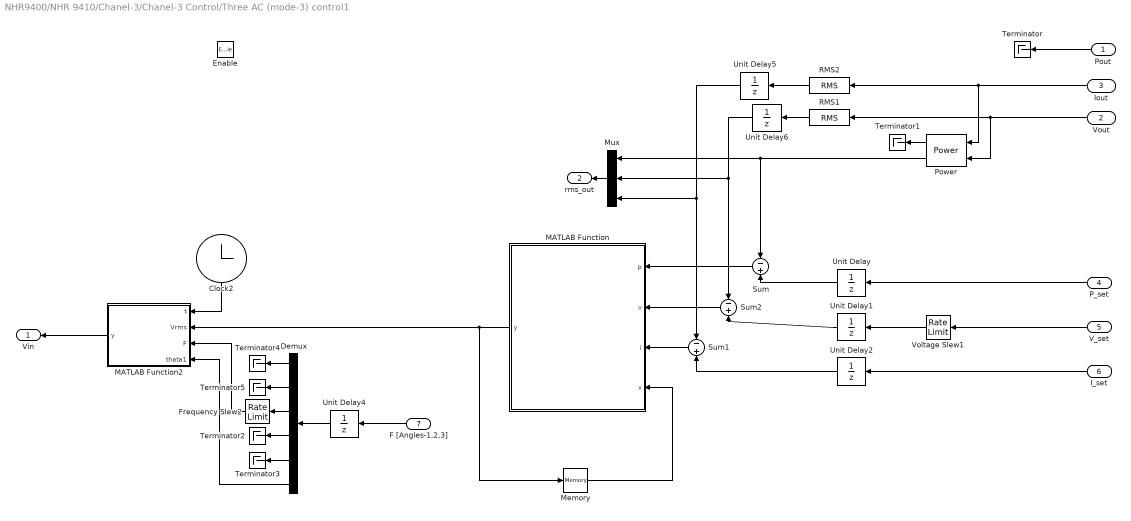
== system NHR9400/NHR 9410/Chanel-3/Chanel-3 Control/Three AC (mode-3) control1 ==
  Pout : Inport
  Vout : Inport  Port=2
  Iout : Inport  Port=3
  P_set : Inport  Port=4
  V_set : Inport  Port=5
  I_set : Inport  Port=6
  F [Angles-1,2,3] : Inport  Port=7
  Enable : EnablePort
  Clock2 : Clock
  Demux : Demux  Outputs=6
  Frequency Slew2 : RateLimiter  RisingSlewLimit=FslewAC  FallingSlewLimit=-FslewAC  SampleTimeMode=inherited  LinearizeAsGain=off
  MATLAB Function : MATLAB Function  TreatAsAtomicUnit=on
  MATLAB Function2 : MATLAB Function  TreatAsAtomicUnit=on
  Memory : Memory
  Mux : Mux  Inputs=3
  Power : powerlib_meascontrol/Measurements/Power  Freq=60  Vinit=[0, 0]  Iinit=[0, 0]  Ts=0
  RMS1 : powerlib_meascontrol/Measurements/RMS  TrueRMS=on  Freq=60  RMSInit=0  Ts=0
  RMS2 : powerlib_meascontrol/Measurements/RMS  TrueRMS=on  Freq=60  RMSInit=0  Ts=0
  Sum : Sum  Inputs=-+
  Sum1 : Sum  Inputs=-+
  Sum2 : Sum  Inputs=-+
  Terminator{,1..5} (6 alike) : Terminator
  Unit Delay{,1..2,4..6} (6 alike) : UnitDelay  SampleTime=-1  HasFrameUpgradeWarning=on
  Voltage Slew1 : RateLimiter  RisingSlewLimit=VslewAC  FallingSlewLimit=-VslewAC  SampleTimeMode=inherited  LinearizeAsGain=off
  Vin : Outport  VectorParamsAs1DForOutWhenUnconnected=off
  rms_out : Outport  Port=2  VectorParamsAs1DForOutWhenUnconnected=off
  wires:
  MATLAB Function/1(y) -> MATLAB Function2/2(Vrms), Memory/1
  Iout/1 -> RMS2/1, Power/2
  Pout/1 -> Terminator/1
  Power/2 -> Terminator1/1
  Sum/1 -> MATLAB Function/1(p)
  Sum2/1 -> MATLAB Function/2(v)
  Sum1/1 -> MATLAB Function/3(i)
  I_set/1 -> Unit Delay2/1
  P_set/1 -> Unit Delay/1
  RMS1/1 -> Unit Delay6/1
  RMS2/1 -> Unit Delay5/1
  Memory/1 -> MATLAB Function/4(x)
  Clock2/1 -> MATLAB Function2/1(t)
  MATLAB Function2/1(y) -> Vin/1
  Power/1 -> Sum/1, Mux/1
  Mux/1 -> rms_out/1
  F [Angles-1,2,3]/1 -> Unit Delay4/1
  Demux/1 -> Terminator4/1
  Demux/4 -> Terminator2/1
  V_set/1 -> Voltage Slew1/1
  Demux/2 -> Terminator5/1
  Demux/5 -> Terminator3/1
  Demux/3 -> Frequency Slew2/1
  Demux/6 -> MATLAB Function2/4(theta1)
  Frequency Slew2/1 -> MATLAB Function2/3(F)
  Voltage Slew1/1 -> Unit Delay1/1
  Unit Delay/1 -> Sum/2
  Unit Delay1/1 -> Sum2/2
  Unit Delay2/1 -> Sum1/2
  Vout/1 -> RMS1/1, Power/1
  Unit Delay4/1 -> Demux/1
  Unit Delay5/1 -> Sum1/1, Mux/3
  Unit Delay6/1 -> Sum2/1, Mux/2

== matlab function NHR9400/NHR 9410/Chanel-3/Chanel-3 Control/All DC (mode-4) control1/MATLAB Function ==
  data: p input; v input; y output; i input; x input
function y = fcn(p,v,i,x)
tol=1e-3;
gain=1e-4;
Ts=1e-3;
if p<=(-tol)
    y=x-(gain/Ts);
elseif i<=(-tol)
    y=x-(gain/Ts);
elseif v<=(-tol)
    y=x-(gain/Ts);
elseif v>tol;
    y=x+(gain/Ts);
else
    y=0;
end

== matlab function NHR9400/NHR 9410/Chanel-1/Chanel-1 Control/All AC control/MATLAB Function ==
  data: p input; v input; y output; i input; x input
function y = fcn(p,v,i,x)
tol=1e-3;
gain=1e-4;
Ts=1e-3;
if p<=(-tol)
    y=x-(gain/Ts);
elseif i<=(-tol)
    y=x-(gain/Ts);
elseif v<=(-tol)
    y=x-(gain/Ts);
elseif v>tol;
    y=x+(gain/Ts);
else
    y=0;
end

== matlab function NHR9400/NHR 9410/Chanel-3/Chanel-3 Control/Three AC (mode-3) control1/MATLAB Function ==
  data: p input; v input; y output; i input; x input
function y = fcn(p,v,i,x)
tol=1e-3;
gain=1e-4;
Ts=1e-3;
if p<=(-tol)
    y=x-(gain/Ts);
elseif i<=(-tol)
    y=x-(gain/Ts);
elseif v<=(-tol)
    y=x-(gain/Ts);
elseif v>tol;
    y=x+(gain/Ts);
else
    y=0;
end

== matlab function NHR9400/NHR 9410/Chanel-1/Chanel-1 Control/All AC control/MATLAB Function2 ==
  data: t input; y output; Vrms input; F input; theta1 input
function y = fcn(t,Vrms,F,theta1)
y = sqrt(2)*Vrms*sin(2*pi*F*t + theta1*pi/180);

== matlab function NHR9400/NHR 9410/Chanel-1/Chanel-1 Control/All DC control/MATLAB Function ==
  data: p input; v input; y output; i input; x input
function y = fcn(p,v,i,x)
tol=1e-3;
gain=1e-4;
Ts=1e-3;
if p<=(-tol)
    y=x-(gain/Ts);
elseif i<=(-tol)
    y=x-(gain/Ts);
elseif v<=(-tol)
    y=x-(gain/Ts);
elseif v>tol;
    y=x+(gain/Ts);
else
    y=0;
end

== matlab function NHR9400/NHR 9410/Chanel-3/Chanel-3 Control/Three AC (mode-3) control1/MATLAB Function2 ==
  data: t input; y output; Vrms input; F input; theta1 input
function y = fcn(t,Vrms,F,theta1)
y = sqrt(2)*Vrms*sin(2*pi*F*t + theta1*pi/180);

== matlab function NHR9400/NHR 9410/Chanel-2/Chanel-2 Control1/All DC control/MATLAB Function ==
  data: p input; v input; y output; i input; x input
function y = fcn(p,v,i,x)
tol=1e-3;
gain=1e-4;
Ts=1e-3;
if p<=(-tol)
    y=x-(gain/Ts);
elseif i<=(-tol)
    y=x-(gain/Ts);
elseif v<=(-tol)
    y=x-(gain/Ts);
elseif v>tol;
    y=x+(gain/Ts);
else
    y=0;
end

== matlab function NHR9400/NHR 9410/Chanel-2/Chanel-2 Control1/All AC control/MATLAB Function ==
  data: p input; v input; y output; i input; x input
function y = fcn(p,v,i,x)
tol=1e-3;
gain=1e-4;
Ts=1e-3;
if p<=(-tol)
    y=x-(gain/Ts);
elseif i<=(-tol)
    y=x-(gain/Ts);
elseif v<=(-tol)
    y=x-(gain/Ts);
elseif v>tol;
    y=x+(gain/Ts);
else
    y=0;
end

== matlab function NHR9400/NHR 9410/Chanel-2/Chanel-2 Control1/All AC control/MATLAB Function2 ==
  data: t input; y output; Vrms input; F input; theta1 input
function y = fcn(t,Vrms,F,theta1)
y = sqrt(2)*Vrms*sin(2*pi*F*t + theta1*pi/180);
